simulink model "InnerLoopMotorKtune"  (R2023b)
settings: Solver=VariableStepAuto  StartTime=0.0  StopTime=100  RelTol=1e-3
model workspace (MAT data in the model file):
  K_in = 1120.00158266
values from neighbouring files (symbols this model uses):
  Js = 0.05116    [Attitude_OuterLoop.m]    (also in BLDC_measures.m; SystemVariables.m)
  Jw = J    (= 0.00254)    [Attitude_OuterLoop.m]    (also in BLDC_measures.m; SystemVariables.m)
  Ke = 67.5e-3    (= 0.0675)    [Attitude_OuterLoop.m]    (also in BLDC_measures.m; SystemVariables.m)
  Kt = Ke    (= 0.0675)    [Attitude_OuterLoop.m]    (also in BLDC_measures.m; SystemVariables.m)
  R = 5.6    [Attitude_OuterLoop.m]    (also in BLDC_measures.m; SystemVariables.m)
libraries: slpidlib x2
settings Model: Creator=Jorge CM  LastModifiedBy=Jorge CM

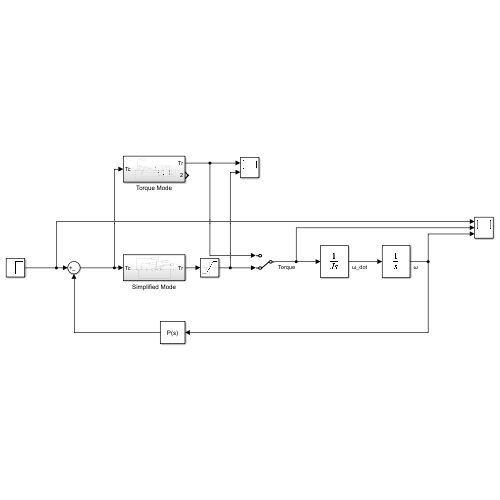
[thumbnail: Simulink's stored preview of the top-level diagram]
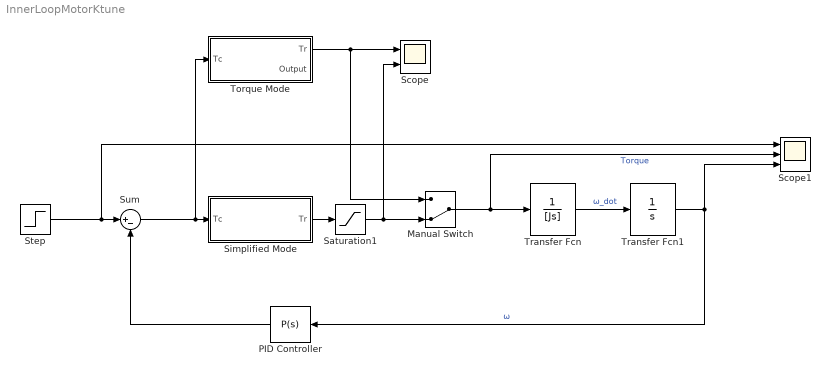
== system InnerLoopMotorKtune ==
  Manual Switch : ManualSwitch  CurrentSetting=0
  PID Controller : slpidlib/PID Controller  Controller=P  Form=Parallel  TimeDomain=Continuous-time  UseExternalTs=off  SampleTime=-1  IntegratorMethod=Forward Euler  FilterMethod=Forward Euler  ControllerParametersSource=internal  P=1  I=1  UseKiTs=off  D=0  N=100  UseFilter=on  TunerSelectOption=Transfer Function Based (PID Tuner App)  InitialConditionSource=internal  InitialConditionForIntegrator=0  InitialConditionForFilter=0  DifferentiatorICPrevScaledInput=0  ExternalReset=none  TrackingMode=off  Kt=1  LimitOutput=off  SatLimitsSource=internal  UpperSaturationLimit=inf  LowerSaturationLimit=-inf  LinearizeAsGain=on  AntiWindupMode=none  Kb=1  LimitIntegrator=off  UpperIntegratorSaturationLimit=inf  LowerIntegratorSaturationLimit=-inf  POutMin=[]  POutMax=[]  IOutMin=[]  IOutMax=[]  DOutMin=[]  DOutMax=[]  NOutMin=[]  NOutMax=[]  SumOutMin=[]  SumOutMax=[]  SaturationOutMin=[]  SaturationOutMax=[]  PParamMin=[]  PParamMax=[]  IParamMin=[]  IParamMax=[]  DParamMin=[]  DParamMax=[]  NParamMin=[]  NParamMax=[]  KbParamMin=[]  KbParamMax=[]  KtParamMin=[]  KtParamMax=[]  KbOutMin=[]  KbOutMax=[]  KtOutMin=[]  KtOutMax=[]  IntegratorOutMin=[]  IntegratorOutMax=[]  FilterOutMin=[]  FilterOutMax=[]  SumI1OutMin=[]  SumI1OutMax=[]  SumI2OutMin=[]  SumI2OutMax=[]  SumI3OutMin=[]  SumI3OutMax=[]  SumI4OutMin=[]  SumI4OutMax=[]  SumDOutMin=[]  SumDOutMax=[]  DifferentiatorOutMin=[]  DifferentiatorOutMax=[]  FilterDiffOutCoefMin=[]  FilterDiffOutCoefMax=[]  ReciprocalOutMin=[]  ReciprocalOutMax=[]  SumDenOutMin=[]  SumDenOutMax=[]  SumNumOutMin=[]  SumNumOutMax=[]  DivideOutMin=[]  DivideOutMax=[]  UdiffTsProdOutMin=[]  UdiffTsProdOutMax=[]  NTsProdOutMin=[]  NTsProdOutMax=[]  UintegralTsProdOutMin=[]  UintegralTsProdOutMax=[]  UngainTsProdOutMin=[]  UngainTsProdOutMax=[]  ClampingZeroOutDataTypeStr=Inherit: Inherit via back propagation  ClampingZeroOutMin=[]  ClampingZeroOutMax=[]  FilterDenConstantOutDataTypeStr=Inherit: Inherit via back propagation  FilterDenConstantOutMin=[]  FilterDenConstantOutMax=[]  PCopyOutDataTypeStr=Inherit: Inherit via back propagation  PCopyOutMin=[]  PCopyOutMax=[]  NCopyOutDataTypeStr=Inherit: Inherit via back propagation  NCopyOutMin=[]  NCopyOutMax=[]  IntegratorContinuousStateAttributes=''  IntegratorStateMustResolveToSignalObject=off  IntegratorRTWStateStorageClass=Auto  FilterContinuousStateAttributes=''  FilterStateMustResolveToSignalObject=off  FilterRTWStateStorageClass=Auto  ParallelPVariant=InternalParameters  IdealPVariant=Disabled  IVariant=Disabled  DVariant=Disabled  IntegratorVariant=Disabled  SatVariant=Disabled  AWVariant=Disabled  PCopyVariant=Disabled  TRVariant=Disabled  FdbkBlocksVariant=Forward  IdealPFdbkVariant=Disabled  SatFdbkVariant=Disabled  DerivativeFilterVariant=Disabled  NVariant=Disabled  NCopyVariant=Disabled_SignalSpec  FilterICVariant=Disabled  IntegratorICVariant=Disabled  ExternalResetVariant=Disabled  TRSumVariant=Passthrough  SumFdbkVariant=Disabled  SumVariant=Passthrough_P  TsampFilterVariant=InternalTs  TsampNgainVariant=Passthrough  TsampIntegralVariant=Disabled_SignalSpec  ExternalSaturationOutDataTypeStr=Inherit: Same as second input
  Saturation1 : Saturate  UpperLimit=Kt  LowerLimit=-Kt
  Scope : Scope  NumInputPorts=2
  Scope1 : Scope  NumInputPorts=3
  Simplified Mode : Subsystem
  Step : Step  After=10  SampleTime=0
  Sum : Sum  Inputs=|+-
  Torque Mode : Subsystem
  Transfer Fcn : TransferFcn  Denominator=[Js]
  Transfer Fcn1 : TransferFcn  Denominator=[1 0]
  wires:
  Torque Mode/1(Tr) -> Manual Switch/1, Scope/1
  Transfer Fcn/1 -> Transfer Fcn1/1  "ω_dot"
  Transfer Fcn1/1 -> PID Controller/1, Scope1/3  "ω"
  Step/1 -> Scope1/1, Sum/1
  Manual Switch/1 -> Transfer Fcn/1, Scope1/2  "Torque"
  PID Controller/1 -> Sum/2
  Simplified Mode/1(Tr) -> Saturation1/1
  Sum/1 -> Torque Mode/1(Tc), Simplified Mode/1(Tc)
  Saturation1/1 -> Manual Switch/2, Scope/2

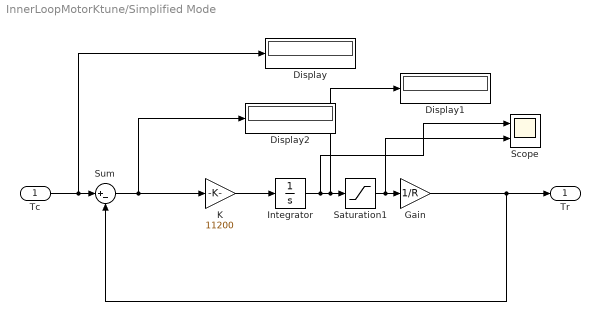
== system InnerLoopMotorKtune/Simplified Mode ==
  Tc : Inport
  Display : Display
  Display1 : Display
  Display2 : Display
  Gain : Gain  Gain=1/R
  Integrator : Integrator
  K : Gain  Gain=11200
  Saturation1 : Saturate  UpperLimit=11  LowerLimit=-11
  Scope : Scope  NumInputPorts=2
  Sum : Sum  Inputs=|+-
  Tr : Outport
  wires:
  K/1 -> Integrator/1
  Tc/1 -> Sum/1, Display/1
  Integrator/1 -> Scope/1, Display1/1, Saturation1/1
  Saturation1/1 -> Scope/2, Gain/1
  Gain/1 -> Tr/1, Sum/2
  Sum/1 -> K/1, Display2/1

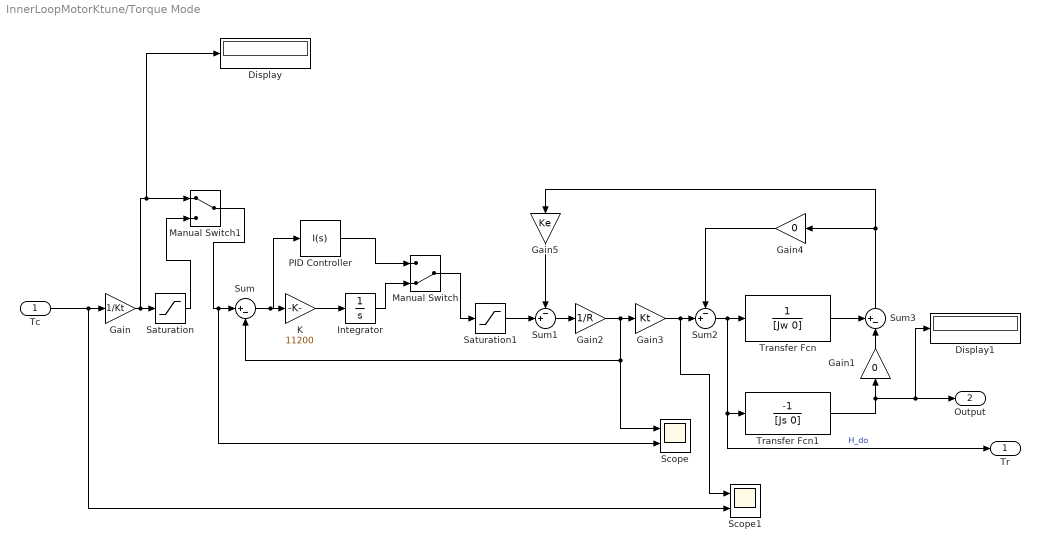
== system InnerLoopMotorKtune/Torque Mode ==
  Tc : Inport
  Display : Display
  Display1 : Display
  Gain : Gain  Gain=1/Kt
  Gain1 : Gain  Gain=0
  Gain2 : Gain  Gain=1/R
  Gain3 : Gain  Gain=Kt
  Gain4 : Gain  Gain=0
  Gain5 : Gain  Gain=Ke
  Integrator : Integrator
  K : Gain  Gain=11200
  Manual Switch : ManualSwitch  CurrentSetting=0
  Manual Switch1 : ManualSwitch
  PID Controller : slpidlib/PID Controller  Controller=I  Form=Parallel  TimeDomain=Continuous-time  UseExternalTs=off  SampleTime=-1  IntegratorMethod=Forward Euler  FilterMethod=Forward Euler  ControllerParametersSource=internal  P=1  I=1120.00158265711  UseKiTs=off  D=0  N=100  UseFilter=on  TunerSelectOption=Transfer Function Based (PID Tuner App)  InitialConditionSource=internal  InitialConditionForIntegrator=0  InitialConditionForFilter=0  DifferentiatorICPrevScaledInput=0  ExternalReset=none  TrackingMode=off  Kt=1  LimitOutput=off  SatLimitsSource=internal  UpperSaturationLimit=inf  LowerSaturationLimit=-inf  LinearizeAsGain=on  AntiWindupMode=none  Kb=1  LimitIntegrator=off  UpperIntegratorSaturationLimit=inf  LowerIntegratorSaturationLimit=-inf  POutMin=[]  POutMax=[]  IOutMin=[]  IOutMax=[]  DOutMin=[]  DOutMax=[]  NOutMin=[]  NOutMax=[]  SumOutMin=[]  SumOutMax=[]  SaturationOutMin=[]  SaturationOutMax=[]  PParamMin=[]  PParamMax=[]  IParamMin=[]  IParamMax=[]  DParamMin=[]  DParamMax=[]  NParamMin=[]  NParamMax=[]  KbParamMin=[]  KbParamMax=[]  KtParamMin=[]  KtParamMax=[]  KbOutMin=[]  KbOutMax=[]  KtOutMin=[]  KtOutMax=[]  IntegratorOutMin=[]  IntegratorOutMax=[]  FilterOutMin=[]  FilterOutMax=[]  SumI1OutMin=[]  SumI1OutMax=[]  SumI2OutMin=[]  SumI2OutMax=[]  SumI3OutMin=[]  SumI3OutMax=[]  SumI4OutMin=[]  SumI4OutMax=[]  SumDOutMin=[]  SumDOutMax=[]  DifferentiatorOutMin=[]  DifferentiatorOutMax=[]  FilterDiffOutCoefMin=[]  FilterDiffOutCoefMax=[]  ReciprocalOutMin=[]  ReciprocalOutMax=[]  SumDenOutMin=[]  SumDenOutMax=[]  SumNumOutMin=[]  SumNumOutMax=[]  DivideOutMin=[]  DivideOutMax=[]  UdiffTsProdOutMin=[]  UdiffTsProdOutMax=[]  NTsProdOutMin=[]  NTsProdOutMax=[]  UintegralTsProdOutMin=[]  UintegralTsProdOutMax=[]  UngainTsProdOutMin=[]  UngainTsProdOutMax=[]  ClampingZeroOutDataTypeStr=Inherit: Inherit via back propagation  ClampingZeroOutMin=[]  ClampingZeroOutMax=[]  FilterDenConstantOutDataTypeStr=Inherit: Inherit via back propagation  FilterDenConstantOutMin=[]  FilterDenConstantOutMax=[]  PCopyOutDataTypeStr=Inherit: Inherit via back propagation  PCopyOutMin=[]  PCopyOutMax=[]  NCopyOutDataTypeStr=Inherit: Inherit via back propagation  NCopyOutMin=[]  NCopyOutMax=[]  IntegratorContinuousStateAttributes=''  IntegratorStateMustResolveToSignalObject=off  IntegratorRTWStateStorageClass=Auto  FilterContinuousStateAttributes=''  FilterStateMustResolveToSignalObject=off  FilterRTWStateStorageClass=Auto  ParallelPVariant=Disabled  IdealPVariant=Disabled  IVariant=InternalParameters  DVariant=Disabled  IntegratorVariant=Continuous  SatVariant=Disabled  AWVariant=Passthrough  PCopyVariant=Disabled  TRVariant=Disabled  FdbkBlocksVariant=Forward  IdealPFdbkVariant=Disabled  SatFdbkVariant=Disabled  DerivativeFilterVariant=Disabled  NVariant=Disabled  NCopyVariant=Disabled_SignalSpec  FilterICVariant=Disabled  IntegratorICVariant=InternalICs  ExternalResetVariant=Disabled  TRSumVariant=Passthrough  SumFdbkVariant=Disabled  SumVariant=Passthrough_I  TsampFilterVariant=InternalTs  TsampNgainVariant=Passthrough  TsampIntegralVariant=Disabled_SignalSpec  ExternalSaturationOutDataTypeStr=Inherit: Same as second input
  Saturation : Saturate  UpperLimit=1  LowerLimit=-1
  Saturation1 : Saturate  UpperLimit=11  LowerLimit=-11
  Scope : Scope  NumInputPorts=2
  Scope1 : Scope  NumInputPorts=2
  Sum : Sum  Inputs=|+-
  Sum1 : Sum  Inputs=-+|
  Sum2 : Sum  Inputs=-+|
  Sum3 : Sum  Inputs=+-|
  Transfer Fcn : TransferFcn  Denominator=[Jw 0]
  Transfer Fcn1 : TransferFcn  Numerator=[-1]  Denominator=[Js 0]
  Tr : Outport
  Output : Outport  Port=2
  wires:
  PID Controller/1 -> Manual Switch/1
  Tc/1 -> Scope1/2, Gain/1
  Manual Switch1/1 -> Scope/2, Sum/1
  Manual Switch/1 -> Saturation1/1
  Transfer Fcn1/1 -> Display1/1, Output/1, Gain1/1
  Sum3/1 -> Gain5/1, Gain4/1
  Gain4/1 -> Sum2/1
  Integrator/1 -> Manual Switch/2
  Sum1/1 -> Gain2/1
  Sum2/1 -> Tr/1, Transfer Fcn1/1, Transfer Fcn/1  "H_do"
  Transfer Fcn/1 -> Sum3/1
  Gain3/1 -> Scope1/1, Sum2/2
  Saturation/1 -> Manual Switch1/2
  Saturation1/1 -> Sum1/2
  Gain2/1 -> Gain3/1, Scope/1, Sum/2
  Sum/1 -> PID Controller/1, K/1
  K/1 -> Integrator/1
  Gain/1 -> Display/1, Manual Switch1/1, Saturation/1
  Gain5/1 -> Sum1/1
  Gain1/1 -> Sum3/2
